simulink model "Attitude_Simulator"  (R2024b)
settings: Solver=VariableStepAuto  StartTime=0.0  StopTime=5  RelTol=1e-3
libraries: simulink_extras x4, sharedtransform x4, aerolibutil x2
settings Model: Creator=waghr  LastModifiedBy=waghr

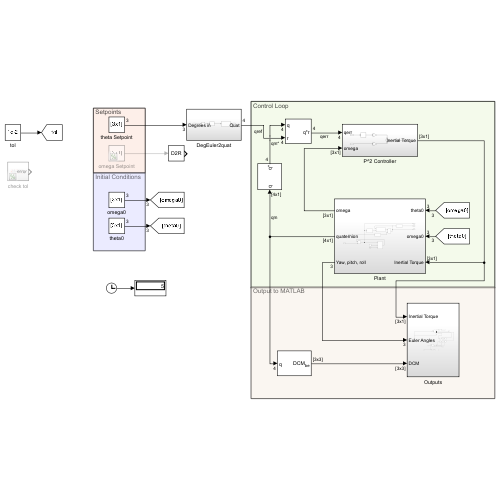
[thumbnail: Simulink's stored preview of the top-level diagram]
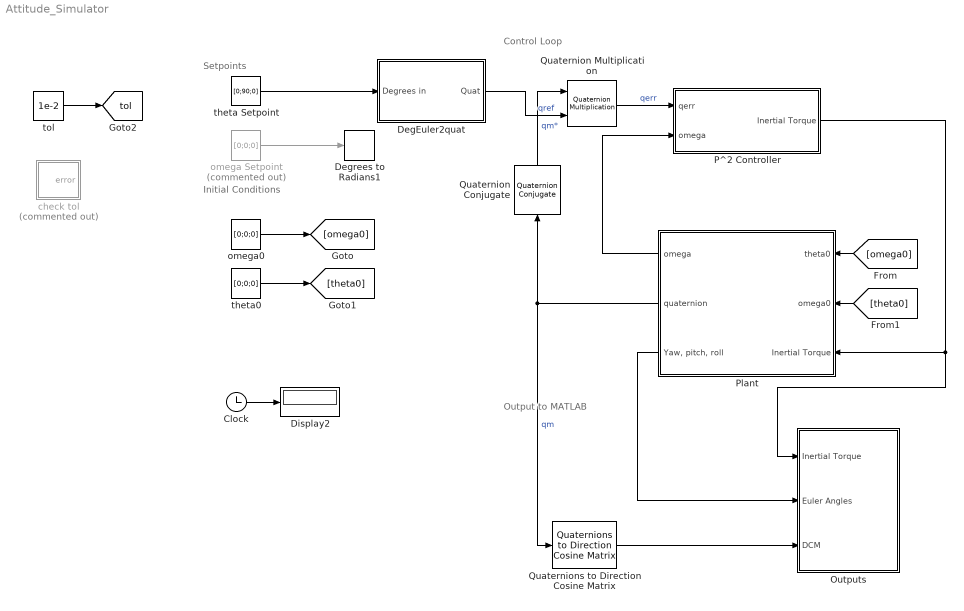
== system Attitude_Simulator ==
  note: Output to MATLAB
  note: Control Loop
  note: Setpoints
  note: Initial Conditions
  Clock : Clock
  DegEuler2quat : Subsystem
  Degrees to Radians1 : simulink_extras/Transformations/Degrees to Radians
  Display2 : Display
  Outputs : Subsystem
  P^2 Controller : Subsystem
  Plant : Subsystem
  Quaternion Conjugate : aerolibutil/Quaternion Conjugate
  Quaternion Multiplication : aerolibutil/Quaternion Multiplication
  Quaternions to Direction Cosine Matrix : sharedtransform/Quaternions to  Direction Cosine Matrix  aMode=aMode
      settings: LibrarySourceBlock=|
      | aerolibtransform2/Quaternions to
      | Direction Cosine Matrix
  check tol : Subsystem  Commented=on
  omega Setpoint : Constant  Commented=on  Value=[0;0;0]
  omega0 : Constant  Value=[0;0;0]
  theta Setpoint : Constant  Value=[0;90;0]
  theta0 : Constant  Value=[0;0;0]
  tol : Constant  Value=1e-2
  tag scope: tol=global
  wires:
  P^2 Controller/1(Inertial Torque) -> Outputs/1(Inertial Torque), Plant/3(Inertial Torque)
  tol/1 -> [tol]
  Clock/1 -> Display2/1
  omega Setpoint/1 -> Degrees to Radians1/1
  Quaternion Multiplication/1 -> P^2 Controller/1(qerr)  "qerr"
  Plant/3("Yaw, pitch, roll") -> Outputs/2(Euler Angles)
  Plant/2(quaternion) -> Quaternions to Direction Cosine Matrix/1, Quaternion Conjugate/1  "qm"
  Quaternions to Direction Cosine Matrix/1 -> Outputs/3(DCM)
  theta Setpoint/1 -> DegEuler2quat/1(Degrees in)
  Quaternion Conjugate/1 -> Quaternion Multiplication/1  "qm*"
  DegEuler2quat/1(Quat) -> Quaternion Multiplication/2  "qref"
  omega0/1 -> [omega0]
  theta0/1 -> [theta0]
  [omega0] -> Plant/1(theta0)
  [theta0] -> Plant/2(omega0)
  Plant/1(omega) -> P^2 Controller/2(omega)

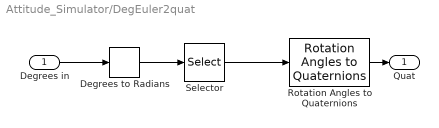
== system Attitude_Simulator/DegEuler2quat ==
  Degrees in : Inport
  Degrees to Radians : simulink_extras/Transformations/Degrees to Radians
  Rotation Angles to Quaternions : sharedtransform/Rotation Angles to Quaternions  rotationOrder=ZYX  aMode=aMode
  Selector : Selector  InputPortWidth=3  IndexOptions=Index vector (dialog)  Indices=[3 2 1]  OutputSizes=1
  Quat : Outport
  wires:
  Rotation Angles to Quaternions/1 -> Quat/1
  Degrees in/1 -> Degrees to Radians/1
  Degrees to Radians/1 -> Selector/1
  Selector/1 -> Rotation Angles to Quaternions/1

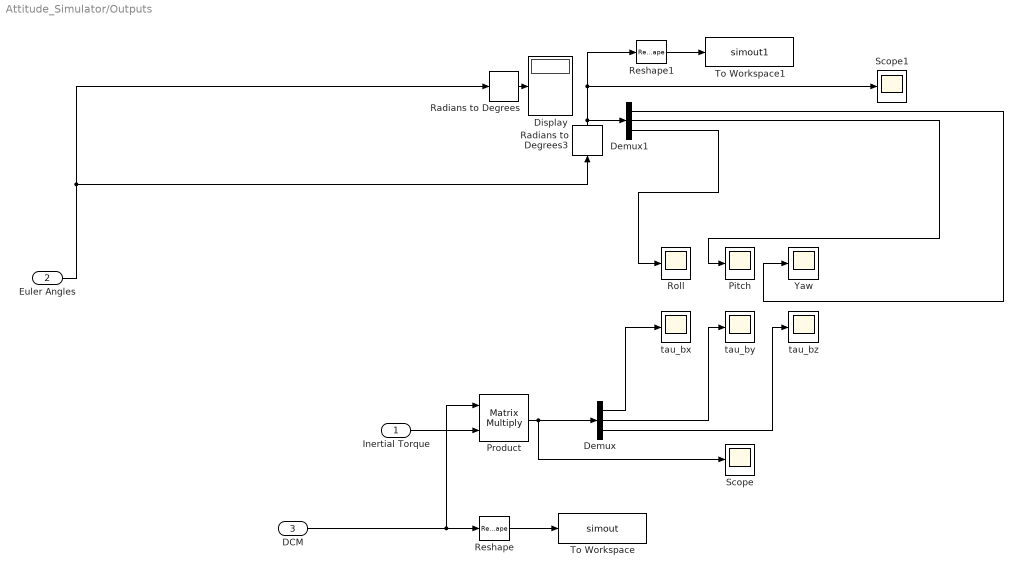
== system Attitude_Simulator/Outputs ==
  Inertial Torque : Inport
  Euler Angles : Inport  Port=2
  DCM : Inport  Port=3
  Demux : Demux  Outputs=3
  Demux1 : Demux  Outputs=3
  Display : Display
  Pitch : Scope
  Product : Product  Multiplication=Matrix(*)
  Radians to Degrees : simulink_extras/Transformations/Radians to Degrees
  Radians to Degrees3 : simulink_extras/Transformations/Radians to Degrees
  Reshape : Reshape
  Reshape1 : Reshape
  Roll : Scope
  Scope : Scope
  Scope1 : Scope
  To Workspace : ToWorkspace  VariableName=simout  SaveFormat=Timeseries  SampleTime=-1
  To Workspace1 : ToWorkspace  VariableName=simout1  SaveFormat=Timeseries  SampleTime=-1
  Yaw : Scope
  tau_bx : Scope
  tau_by : Scope
  tau_bz : Scope
  wires:
  DCM/1 -> Product/1, Reshape/1
  Radians to Degrees3/1 -> Scope1/1, Reshape1/1, Demux1/1
  Reshape1/1 -> To Workspace1/1
  Demux1/1 -> Yaw/1
  Demux/3 -> tau_bz/1
  Inertial Torque/1 -> Product/2
  Demux/2 -> tau_by/1
  Demux1/2 -> Pitch/1
  Euler Angles/1 -> Radians to Degrees3/1, Radians to Degrees/1
  Demux1/3 -> Roll/1
  Reshape/1 -> To Workspace/1
  Product/1 -> Scope/1, Demux/1
  Demux/1 -> tau_bx/1
  Radians to Degrees/1 -> Display/1

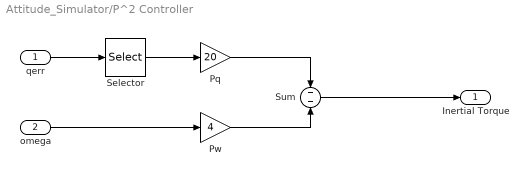
== system Attitude_Simulator/P^2 Controller ==
  qerr : Inport
  omega : Inport  Port=2
  Pq : Gain  Gain=20
  Pw : Gain  Gain=4
  Selector : Selector  InputPortWidth=4  IndexOptions=Index vector (dialog)  Indices=[2 3 4]  OutputSizes=1
  Sum : Sum  Inputs=--
  Inertial Torque : Outport
  wires:
  Sum/1 -> Inertial Torque/1
  qerr/1 -> Selector/1
  omega/1 -> Pw/1
  Pw/1 -> Sum/2
  Pq/1 -> Sum/1
  Selector/1 -> Pq/1

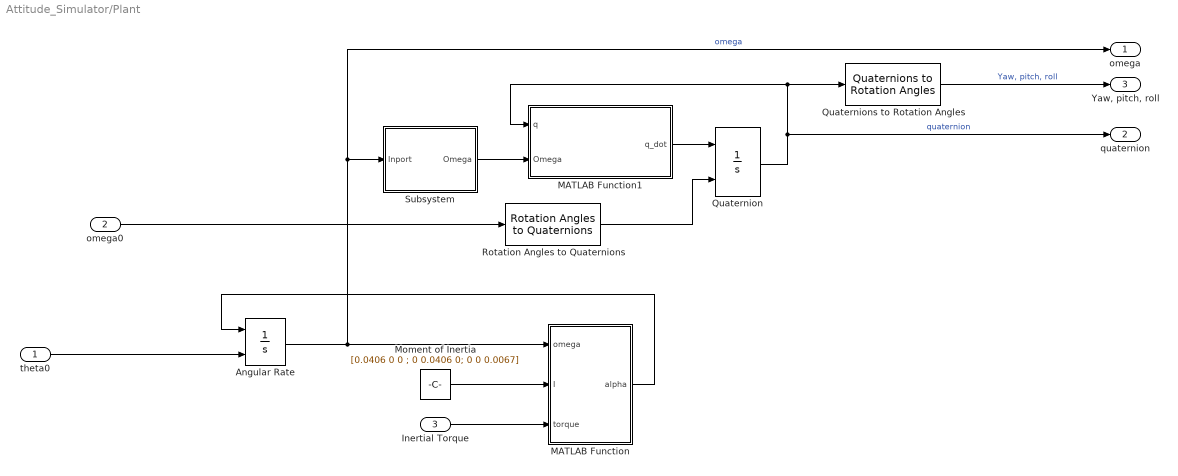
== system Attitude_Simulator/Plant ==
  theta0 : Inport
  omega0 : Inport  Port=2
  Inertial Torque : Inport  Port=3
  Angular Rate : Integrator  InitialConditionSource=external
  MATLAB Function : MATLAB Function  TreatAsAtomicUnit=on
  MATLAB Function1 : MATLAB Function  TreatAsAtomicUnit=on
  Moment of Inertia : Constant  Value=[0.0406 0 0 ; 0 0.0406 0; 0 0 0.0067]
  Quaternion : Integrator  InitialConditionSource=external  InitialCondition=[1;0;0;0]
  Quaternions to Rotation Angles : sharedtransform/Quaternions to Rotation Angles  rotationOrder=ZYX  aMode=aMode
  Rotation Angles to Quaternions : sharedtransform/Rotation Angles to Quaternions  rotationOrder=ZYX  aMode=aMode
  Subsystem : Subsystem
  omega : Outport
  quaternion : Outport  Port=2
  "Yaw, pitch, roll" : Outport  Port=3
  wires:
  Rotation Angles to Quaternions/1 -> Quaternion/2
  Angular Rate/1 -> MATLAB Function/1(omega), Subsystem/1(Inport), omega/1  "omega"
  Inertial Torque/1 -> MATLAB Function/3(torque)
  Subsystem/1(Omega) -> MATLAB Function1/2(Omega)
  Moment of Inertia/1 -> MATLAB Function/2(I)
  MATLAB Function1/1(q_dot) -> Quaternion/1
  MATLAB Function/1(alpha) -> Angular Rate/1
  Quaternion/1 -> Quaternions to Rotation Angles/1, MATLAB Function1/1(q), quaternion/1  "quaternion"
  omega0/1 -> Rotation Angles to Quaternions/1
  theta0/1 -> Angular Rate/2
  Quaternions to Rotation Angles/1 -> "Yaw, pitch, roll"/1  "Yaw, pitch, roll"

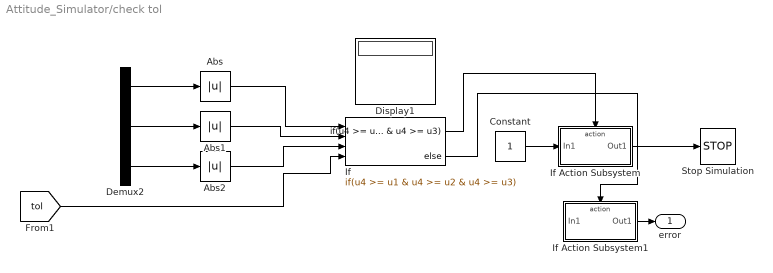
== system Attitude_Simulator/check tol ==
  Abs : Abs  SaturateOnIntegerOverflow=off
  Abs1 : Abs  SaturateOnIntegerOverflow=off
  Abs2 : Abs  SaturateOnIntegerOverflow=off
  Constant : Constant
  Demux2 : Demux  Outputs=3
  Display1 : Display
  If : If  NumInputs=4  IfExpression=u4 >= u1 & u4 >= u2 & u4 >= u3
  If Action Subsystem : Subsystem  TreatAsAtomicUnit=on
  If Action Subsystem1 : Subsystem  TreatAsAtomicUnit=on
  Stop Simulation : Stop
  error : Outport
  wires:
  Demux2/3 -> Abs2/1
  ? -> If Action Subsystem1/1(In1), Display1/1, Demux2/1
  If/1 -> If Action Subsystem/Action
  Constant/1 -> If Action Subsystem/1(In1)
  Demux2/2 -> Abs1/1
  If Action Subsystem/1(Out1) -> Stop Simulation/1
  If/2 -> If Action Subsystem1/Action
  Abs/1 -> If/1
  [tol] -> If/4
  Abs1/1 -> If/2
  Abs2/1 -> If/3
  Demux2/1 -> Abs/1
  If Action Subsystem1/1(Out1) -> error/1

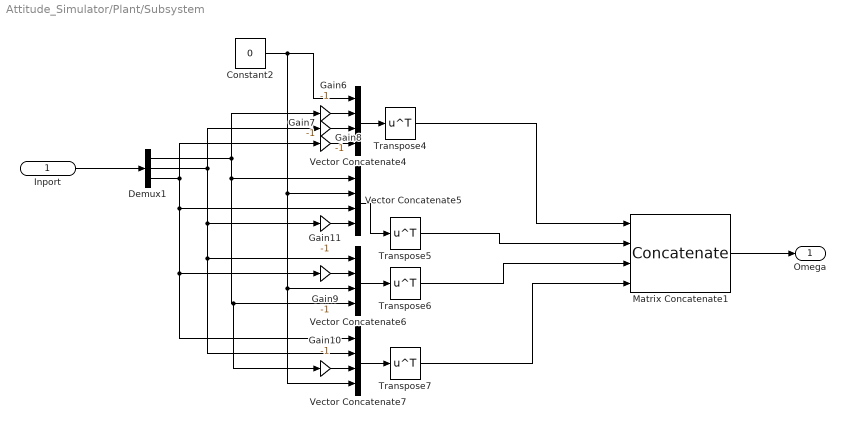
== system Attitude_Simulator/Plant/Subsystem ==
  Inport : Inport
  Constant2 : Constant  Value=0
  Demux1 : Demux  Outputs=3
  Gain{6..11} (6 alike) : Gain  Gain=-1
  Matrix Concatenate1 : Concatenate  NumInputs=4  Mode=Multidimensional array
  Transpose{4..7} (4 alike) : Math  Operator=transpose
  Vector Concatenate{4..7} (4 alike) : Concatenate  NumInputs=4
  Omega : Outport
  wires:
  Gain11/1 -> Vector Concatenate5/4
  Gain8/1 -> Vector Concatenate4/4
  Transpose4/1 -> Matrix Concatenate1/1
  Transpose7/1 -> Matrix Concatenate1/4
  Vector Concatenate5/1 -> Transpose5/1
  Vector Concatenate6/1 -> Transpose6/1
  Transpose5/1 -> Matrix Concatenate1/2
  Inport/1 -> Demux1/1
  Demux1/1 -> Gain10/1, Vector Concatenate6/4, Vector Concatenate5/1, Gain6/1
  Vector Concatenate4/1 -> Transpose4/1
  Demux1/3 -> Vector Concatenate5/3, Vector Concatenate7/1, Gain9/1, Gain8/1
  Gain7/1 -> Vector Concatenate4/3
  Demux1/2 -> Vector Concatenate7/2, Vector Concatenate6/1, Gain11/1, Gain7/1
  Gain9/1 -> Vector Concatenate6/2
  Transpose6/1 -> Matrix Concatenate1/3
  Constant2/1 -> Vector Concatenate7/4, Vector Concatenate6/3, Vector Concatenate5/2, Vector Concatenate4/1
  Vector Concatenate7/1 -> Transpose7/1
  Gain6/1 -> Vector Concatenate4/2
  Gain10/1 -> Vector Concatenate7/3
  Matrix Concatenate1/1 -> Omega/1

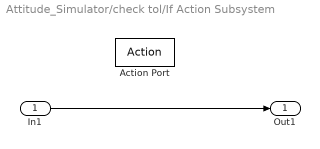
== system Attitude_Simulator/check tol/If Action Subsystem ==
  In1 : Inport
  Action Port : ActionPort  ActionPortLabel=if(u4 >= u1 & u4 >= u2 & u4 >= u3)
  Out1 : Outport
  wires:
  In1/1 -> Out1/1

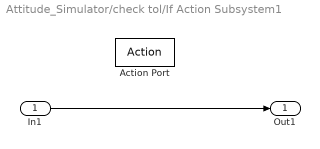
== system Attitude_Simulator/check tol/If Action Subsystem1 ==
  In1 : Inport
  Action Port : ActionPort  ActionPortLabel=else
  Out1 : Outport
  wires:
  In1/1 -> Out1/1

== matlab function Attitude_Simulator/Plant/MATLAB Function1 ==
  data: q input; Omega input; q_dot output
function q_dot = qKinematics(q,Omega)
q_dot = 0.5 * Omega * q;
end

== matlab function Attitude_Simulator/Plant/MATLAB Function ==
  data: alpha output; omega input; I input; torque input
function alpha = getAlpha(omega, I, torque)
    % omega: [3x1] angular velocity
    % I: [3x3] inertia matrix
    % torque: [3x1] applied torque
    alpha = I \ (torque - cross(omega, I * omega));
end
